simulink model "Main_model"  (R2021b)
settings: Solver=ode23t  StartTime=0.0  StopTime=sim_t_end  RelTol=1e-3
undefined symbols (not defined in the file): ambient_co2, ambient_pressure, ambient_rh, ambient_temp, battery, battery_heat_gen_scale, battery_mass, battery_thermal_mass, cab_air_v_dot, cabin_heater_cmd, cabin_heater_max_power, case_cold_plate_mass, case_cold_plate_thermal_mass, chiller_baffles_n, chiller_tube_length, chiller_tubes_n_rows, compressor_max_m_dot, compressor_ref_m_dot, condenser_air_min_flow_area, condenser_tube_width, const_current, coolant_channel_length, coolant_initial_T, coolant_m_dot, coolant_pipe_cross_sec_area, evaporator_air_cross_sec_area, evaporator_air_min_flow_area, evaporator_tube_width, motor_mc_heat_fraction, n_parallel, power_fraction_rear, ptc_heater_max_power, ptc_heater_thermal_mass, rad_air_v_dot, radiator_air_cross_sec_area, radiator_air_min_flow_area, radiator_tube_width, ref_m_dot, ref_pipe_dia, refrigerant_initial_void_fraction, refrigerant_pipe_cross_sec_area, T_bat_active_cool, T_bat_active_heat, T_bat_passive_cool, T_bat_passive_heat, T_battery_init, T_battery_nom, T_cabin_init, T_cabin_setpoint, T_dcdc_nom, T_DT_high, T_DT_passive_cool, T_DT_whr_active, T_front_gb_nom, T_front_mc_nom, T_front_motor_nom, T_rear_gb_nom, T_rear_mc_nom, T_rear_motor_nom, three_w_valve_max_open_area_factor ... (+3)
libraries: fl_lib x448, nesl_utility x328, SimscapeFluids_lib x134, slpidlib x15, ee_lib x9, simulink x8, LiBatteryElements_lib x4, SignalEditorBlockLib x1
(part 11 of 24)

== system Main_model/HVAC cycles/4 Way Valve (2P)2 ==
  Orifice (2P){6..9} (4 alike) : SimscapeFluids_lib/Two-Phase Fluid/Valves & Orifices/Orifice (2P)  orifice_type=foundation.enum.constant_variable.variable  mdot_nominal_constant=0.1 kg/s  delta_p_nominal_constant=0.001 MPa  S_min=0 m  del_S=5e-3 m  open_orientation=fluids.two_phase_fluid.valves_orifices.enum.OrificeOrientation.Positive  mdot_nominal_max=0.018 kg/s  delta_p_nominal_max=0.001 MPa  energy_spec=foundation.enum.energy_spec.void_fraction  p_inlet=.7 MPa  T_inlet=293.15 K  x_inlet=0.5  alpha_inlet=refrigerant_initial_void_fraction  h_inlet=1500 kJ/kg  u_inlet=1500 kJ/kg  area=refrigerant_pipe_cross_sec_area m^2  mdot_leak_fraction=1e-6  smoothing_factor=0.01  B_lam=0.999  tau_x=0.1 s
      settings: SourceProductBaseCode=SH  InternalSimscapePortConfiguration="{\"Bottom\":[],\"Left\":[{\"id\":\"A\",\"label\":\"A\",\"type\":\"foundation.two_phase_fluid.two_phase_fluid\"},{\"id\":\"S\",\"label\":\"S\",\"type\":\"input\"}],\"Right\":[{\"id\":\"B\",\"label\":\"B\",\"type\":\"foundation.two_phase_fluid.two_phase_fluid\"}],\"Top\":[]}"
  PS Gain : fl_lib/Physical Signals/Functions/PS Gain  gain=-1
  Simulink-PS Converter : nesl_utility/Simulink-PS Converter  PhysicalDomain=network_engine_domain  SubClassName=ps_input  LeftPortType=input  RightPortType=output  PseudoPeriodic=off  Frequencies=[]  NoiseDistribution=none  NoiseParameters=[]  Unit=1  AffineConversion=off  FilteringAndDerivatives=provide  SimscapeFilterOrder=1  InputFilterTimeConstant=0.001  UdotUserProvided=0
      settings: SourceProductBaseCode=PW,SS
  A1 : PMIOPort  Side=Left
  A2 : PMIOPort  Port=2  Side=Right
  B2 : PMIOPort  Port=3  Side=Left
  B1 : PMIOPort  Port=4  Side=Right
  wires:
  [cmd_cool_heat_loop] -> Simulink-PS Converter/1
  connections:
  B2/RConn1 -- Orifice (2P)8/LConn1 -- Orifice (2P)9/RConn1
  Orifice (2P)9/LConn2 -- PS Gain/LConn1 -- Orifice (2P)6/LConn2 -- Simulink-PS Converter/RConn1
  A2/RConn1 -- Orifice (2P)7/LConn1 -- Orifice (2P)6/RConn1
  A1/RConn1 -- Orifice (2P)6/LConn1 -- Orifice (2P)8/RConn1
  B1/RConn1 -- Orifice (2P)7/RConn1 -- Orifice (2P)9/LConn1
  Orifice (2P)8/LConn2 -- PS Gain/RConn1 -- Orifice (2P)7/LConn2

== system Main_model/HVAC cycles/4 Way Valve (2P)3 ==
  Orifice (2P){6..9} (4 alike) : SimscapeFluids_lib/Two-Phase Fluid/Valves & Orifices/Orifice (2P)  orifice_type=foundation.enum.constant_variable.variable  mdot_nominal_constant=0.1 kg/s  delta_p_nominal_constant=0.001 MPa  S_min=0 m  del_S=5e-3 m  open_orientation=fluids.two_phase_fluid.valves_orifices.enum.OrificeOrientation.Positive  mdot_nominal_max=0.018 kg/s  delta_p_nominal_max=0.001 MPa  energy_spec=foundation.enum.energy_spec.void_fraction  p_inlet=.7 MPa  T_inlet=293.15 K  x_inlet=0.5  alpha_inlet=refrigerant_initial_void_fraction  h_inlet=1500 kJ/kg  u_inlet=1500 kJ/kg  area=refrigerant_pipe_cross_sec_area m^2  mdot_leak_fraction=1e-6  smoothing_factor=0.01  B_lam=0.999  tau_x=0.1 s
      settings: SourceProductBaseCode=SH  InternalSimscapePortConfiguration="{\"Bottom\":[],\"Left\":[{\"id\":\"A\",\"label\":\"A\",\"type\":\"foundation.two_phase_fluid.two_phase_fluid\"},{\"id\":\"S\",\"label\":\"S\",\"type\":\"input\"}],\"Right\":[{\"id\":\"B\",\"label\":\"B\",\"type\":\"foundation.two_phase_fluid.two_phase_fluid\"}],\"Top\":[]}"
  PS Gain : fl_lib/Physical Signals/Functions/PS Gain  gain=-1
  Simulink-PS Converter : nesl_utility/Simulink-PS Converter  PhysicalDomain=network_engine_domain  SubClassName=ps_input  LeftPortType=input  RightPortType=output  PseudoPeriodic=off  Frequencies=[]  NoiseDistribution=none  NoiseParameters=[]  Unit=1  AffineConversion=off  FilteringAndDerivatives=provide  SimscapeFilterOrder=1  InputFilterTimeConstant=0.001  UdotUserProvided=0
      settings: SourceProductBaseCode=PW,SS
  A1 : PMIOPort  Side=Left
  A2 : PMIOPort  Port=2  Side=Right
  B2 : PMIOPort  Port=3  Side=Left
  B1 : PMIOPort  Port=4  Side=Right
  wires:
  [cmd_cool_heat_loop] -> Simulink-PS Converter/1
  connections:
  B2/RConn1 -- Orifice (2P)8/LConn1 -- Orifice (2P)9/RConn1
  Orifice (2P)9/LConn2 -- PS Gain/LConn1 -- Orifice (2P)6/LConn2 -- Simulink-PS Converter/RConn1
  A2/RConn1 -- Orifice (2P)7/LConn1 -- Orifice (2P)6/RConn1
  A1/RConn1 -- Orifice (2P)6/LConn1 -- Orifice (2P)8/RConn1
  B1/RConn1 -- Orifice (2P)7/RConn1 -- Orifice (2P)9/LConn1
  Orifice (2P)8/LConn2 -- PS Gain/RConn1 -- Orifice (2P)7/LConn2

== system Main_model/HVAC cycles/Compressor On-Off ==
  1-D Lookup Table : Lookup_n-D  NumberOfTableDimensions=1  BreakpointsForDimension1=[0,.03,0.05,0.1,0.15,0.2,0.25,0.3,1]  Table=[0,0,0.1*compressor_ref_m_dot,0.3*compressor_ref_m_dot,0.4*compressor_ref_m_dot,0.5*compressor_ref_m_dot,0.7*compressor_ref_m_dot,compressor_ref_m_dot,compressor_ref_m_dot]  InternalRulePriority=Speed  RndMeth=Simplest  InputSameDT=on
  1-D Lookup Table1 : Lookup_n-D  NumberOfTableDimensions=1  BreakpointsForDimension1=[0.5,0.7,1,2,3,4,5,5.5]  Table=[compressor_ref_m_dot,compressor_ref_m_dot,compressor_ref_m_dot,.7*compressor_ref_m_dot,.2*compressor_ref_m_dot,.005*compressor_ref_m_dot,0,0]  InternalRulePriority=Speed  RndMeth=Simplest  InputSameDT=on
  Constant : Constant  Value=ambient_temp
  Constant1 : Constant  Commented=on  Value=.0001
  Constant2 : Constant  Value=T_cabin_setpoint
  Constant3 : Constant  Value=0
  Constant4 : Constant  Commented=on  Value=.05
  Constant5 : Constant
  Constant6 : Constant  Value=0
  Constant7 : Constant  Value=-1
  Constant8 : Constant
  Data Type Conversion1 : DataTypeConversion
  Data Type Conversion3 : DataTypeConversion
  Data Type Conversion4 : DataTypeConversion  Commented=on
  Delay : Delay  Commented=on  DelayLength=10
  Delay1 : Delay  Commented=on  DelayLength=10
  Gain : Gain  Gain=1/compressor_ref_m_dot
  Gain1 : Gain  Gain=60*5/18
  GreaterThan : RelationalOperator  Commented=on  Operator=>  OutDataTypeStr=boolean  RndMeth=Simplest
  GreaterThan1 : RelationalOperator  Operator=>  OutDataTypeStr=boolean  RndMeth=Simplest
  GreaterThan2 : RelationalOperator  Operator=<  OutDataTypeStr=boolean  RndMeth=Simplest
  GreaterThan3 : RelationalOperator  Operator=>  OutDataTypeStr=boolean  RndMeth=Simplest
  Min : MinMax  Inputs=2
  Mux : Mux  Inputs=2
  Mux1 : Mux  Inputs=3
  Relay1 : Relay  OnSwitchValue=T_cabin_setpoint+2  OffSwitchValue=T_cabin_setpoint-2  OnOutputValue=1.1*T_cabin_setpoint  OffOutputValue=0.9*T_cabin_setpoint
  Relay2 : Relay  OnSwitchValue=T_cabin_setpoint+2  OffSwitchValue=T_cabin_setpoint-2  OnOutputValue=1.1*T_cabin_setpoint  OffOutputValue=0.9*T_cabin_setpoint
  Scope : Scope  NumInputPorts=2
  Scope2 : Scope  NumInputPorts=2
  Step : Step  SampleTime=0
  Step1 : Step  SampleTime=0
  Switch{1..3,5} (4 alike) : Switch  Criteria=u2 > Threshold  OutDataTypeStr=double
  Switch4 : Switch  Commented=on  Criteria=u2 > Threshold  OutDataTypeStr=double
  Transfer Fcn1 : TransferFcn  Commented=on  Denominator=[.1 1]
  Transfer Fcn2 : TransferFcn  Denominator=[.5 1]
  tag scope: ac_onoff=global, cmd_compressor_m_dot=global, cmd_cool_heat_loop=global, cmd_hvac_pump_on_off=global, hvac_cmd_fan=global, veh_speed_m_s=global
  wires:
  Data Type Conversion1/1 -> Switch5/2, Switch1/2
  GreaterThan1/1 -> Switch2/1
  Constant3/1 -> Switch1/3
  Constant2/1 -> GreaterThan3/2, Mux1/2, GreaterThan1/2, GreaterThan2/2  "T setpoint"
  Switch2/1 -> Data Type Conversion1/1
  Constant/1 -> Mux1/3, GreaterThan3/1  "T ambient"
  GreaterThan2/1 -> Switch2/3
  GreaterThan3/1 -> Data Type Conversion3/1, Switch2/2
  [T_cabin] -> Relay1/1, Delay1/1, Mux1/1, Relay2/1  "T cabin"
  Transfer Fcn2/1 -> GreaterThan/1, Scope2/1, [cmd_compressor_m_dot], Gain/1  "cmd_compressor_m_dot"
  1-D Lookup Table/1 -> Min/1
  1-D Lookup Table1/1 -> Min/2
  [p_evap_comp_in] -> 1-D Lookup Table/1
  [p_cond_comp_in] -> 1-D Lookup Table1/1
  Min/1 -> Transfer Fcn2/1, Switch1/1
  Switch3/1 -> Mux/1, [cmd_cool_heat_loop]  "cmd cooling (1) or heating (-1) mode (4-way valve)"
  Constant7/1 -> Switch3/3
  Data Type Conversion3/1 -> Switch3/1, Switch3/2
  Gain/1 -> Mux/2  "cmd compressor refrigerant mass flow rate"
  Mux/1 -> Scope/2
  Mux1/1 -> Scope/1
  Constant1/1 -> GreaterThan/2
  GreaterThan/1 -> Switch4/2, Data Type Conversion4/1
  Data Type Conversion4/1 -> Switch4/1
  Switch4/1 -> Scope2/2, Transfer Fcn1/1  "cmd_hvac_pump_on_off"
  Constant4/1 -> Switch4/3
  Constant5/1 -> [cmd_hvac_pump_on_off]  "cmd_compressor_m_dot"
  Constant6/1 -> Switch5/3
  Constant8/1 -> Switch5/1
  Switch5/1 -> [ac_onoff]
  Relay2/1 -> GreaterThan1/1
  Relay1/1 -> GreaterThan2/1
  Step/1 -> [hvac_cmd_fan]
  Gain1/1 -> [veh_speed_m_s]
  Step1/1 -> Gain1/1

== system Main_model/HVAC cycles/LCC4 ==
  lcc : SimscapeFluids_lib/Fluid Network Interfaces/Heat Exchangers/Condenser Evaporator (TL-2P)  flow_arrangement=fluids.interfaces.heat_exchangers.enum.FlowArrangementTL2P.Cross  cross_flow_arrangement=fluids.interfaces.heat_exchangers.enum.CrossFlowArrangementTL2P.UnmixedMixed  R_wall=chiller_wall_thermal_resistance K/kW  area_A1=coolant_pipe_cross_sec_area m^2  area_B1=coolant_pipe_cross_sec_area m^2  area_A2=refrigerant_pipe_cross_sec_area m^2  area_B2=refrigerant_pipe_cross_sec_area m^2  flow_geometry_TL=fluids.interfaces.heat_exchangers.enum.FlowGeometryTL.AcrossTubeBank  tube_num_TL=25  tube_length_TL=1 m  tube_cross_section_TL=fluids.interfaces.heat_exchangers.enum.TubeCrossSection.Rectangular  tube_diameter_TL=0.05 m  tube_width_TL=.02 m  tube_height_TL=0.003 m  tube_inner_diameter_TL=0.05 m  tube_outer_diameter_TL=0.1 m  tube_flow_area_TL=0.002 m^2  tube_wetted_perimeter_TL=0.15 m  tube_heat_perimeter_TL=0.15 m  tube_pressure_loss_spec_TL=fluids.interfaces.heat_exchangers.enum.TubePressureLossSpec.Haaland  tube_loss_coeff_TL=10  tube_length_add_TL=4 m  tube_roughness_pressure_TL=15e-6 m  tube_Re_lam_pressure_TL=2000  tube_Re_tur_pressure_TL=4000  tube_shape_factor_generic_TL=64  tube_heat_coeff_spec_TL=fluids.interfaces.heat_exchangers.enum.TubeHeatCoeffSpec.Gneilinski  tube_colburn_coeff_TL=[.023, .8, .33]  tube_roughness_heat_TL=15e-6 m  tube_Re_lam_heat_TL=2000  tube_Re_tur_heat_TL=4000  tube_Nu_lam_generic_TL=3.66  bank_arrangement_TL=fluids.interfaces.heat_exchangers.enum.BankArrangement.Staggered  bank_num_rows_TL=chiller_tubes_n_rows*(chiller_baffles_n+1)  bank_tubes_per_row_TL=chiller_tubes_n_columns  bank_width_TL=chiller_tube_length/(chiller_baffles_n+1) m  bank_tube_diameter_TL=chiller_tube_dia m  bank_longitudinal_pitch_TL=chiller_long_pitch m  bank_transverse_pitch_TL=chiller_transverse_pitch m  bank_pressure_loss_spec_TL=fluids.interfaces.heat_exchangers.enum.BankPressureLossSpec.Euler  bank_euler_TL=70  bank_heat_coeff_spec_TL=fluids.interfaces.heat_exchangers.enum.BankHeatCoeffSpec.Colburn  bank_colburn_coeff_TL=[0.27, .67, 0.36]  generic_flow_area_TL=0.01 m^2  generic_heat_area_TL=2 m^2  generic_volume_TL=0.05 m^3  generic_loss_coeff_TL=10  generic_colburn_coeff_TL=[.023, .8, .33]  fouling_factor_TL=0.1 K*m^2/kW  fin_area_TL=chiller_baffles_area m^2  fin_efficiency_TL=chiller_bafffles_fin_eff  p_init_TL=ambient_pressure MPa  T_init_TL=ambient_temp K  tube_num_2P=chiller_tubes_n_total  tube_length_2P=chiller_tube_length m  tube_cross_section_2P=fluids.interfaces.heat_exchangers.enum.TubeCrossSection.Circular  tube_diameter_2P=chiller_tube_dia m  tube_width_2P=0.05 m  tube_height_2P=0.05 m  tube_inner_diameter_2P=0.05 m  tube_outer_diameter_2P=0.1 m  tube_flow_area_2P=0.002 m^2  tube_wetted_perimeter_2P=0.15 m  tube_heat_perimeter_2P=0.15 m  tube_pressure_loss_spec_2P=fluids.interfaces.heat_exchangers.enum.TubePressureLossSpec2P.LossCoeff  tube_loss_coeff_2P=10  tube_length_add_2P=chiller_tube_eqv_resistance_length m  tube_roughness_pressure_2P=15e-6 m  tube_Re_lam_pressure_2P=2000  tube_Re_tur_pressure_2P=4000  tube_shape_factor_generic_2P=64  tube_heat_coeff_spec_2P=fluids.interfaces.heat_exchangers.enum.TubeHeatCoeffSpec2P.Colburn  tube_colburn_coeff_liq_2P=[0.27, .67, 0.36]  tube_colburn_coeff_mix_2P=[0.27, .67, 0.36]  tube_colburn_coeff_vap_2P=[0.27, .67, 0.36]  tube_roughness_heat_2P=15e-6 m  tube_Re_lam_heat_2P=2000  tube_Re_tur_heat_2P=4000  tube_Nu_lam_generic_2P=3.66  fouling_factor_2P=0.1 K*m^2/kW  fin_area_2P=0 m^2  fin_efficiency_2P=0  energy_spec_2P=foundation.enum.energy_spec.void_fraction  p_init_2P=refrigerant_initial_P MPa  T_init_2P=refrigerant_initial_T K  x_init_2P=0.5  alpha_init_2P=refrigerant_initial_void_fraction  h_init_2P=1500 kJ/kg  u_init_2P=1500 kJ/kg
      settings: SourceProductBaseCode=SH  InternalSimscapePortConfiguration="{\"Bottom\":[],\"Left\":[{\"id\":\"A1\",\"label\":\"A1\",\"type\":\"foundation.thermal_liquid.thermal_liquid\"},{\"id\":\"B1\",\"label\":\"B1\",\"type\":\"foundation.thermal_liquid.thermal_liquid\"}],\"Right\":[{\"id\":\"A2\",\"label\":\"A2\",\"type\":\"foundation.two_phase_fluid.two_phase_fluid\"},{\"id\":\"B2\",\"label\":\"B2\",\"type\":\"foundation.two_phase_fluid.two_phase_fluid\"}],\"Top\":[{\"id\":\"Z\",\"label\":\"Z\",\"type\":\"output\"}]}"
  Coolant Out : PMIOPort  Side=Left
  Coolant In : PMIOPort  Port=2  Side=Left
  Ref In : PMIOPort  Port=3  Side=Right
  Ref Out : PMIOPort  Port=4  Side=Right
  connections:
  lcc/RConn1 -- Ref In/RConn1
  lcc/LConn1 -- Coolant In/RConn1
  lcc/LConn2 -- Coolant Out/RConn1
  lcc/RConn2 -- Ref Out/RConn1

== system Main_model/HVAC cycles/TXV1 ==
  Cap (2P) : fl_lib/Two-Phase Fluid/Elements/Cap (2P)  p_specify=off  p_priority=None  p=0.101325 MPa  p_nominal_specify=off  p_nominal_unit=MPa  p_nominal_value=1  u_specify=off  u_priority=None  u=1.5e+3 kJ/kg  u_nominal_specify=off  u_nominal_unit=kJ/kg  u_nominal_value=1
      settings: SourceProductBaseCode=SS  InternalSimscapePortConfiguration="{\"Bottom\":[],\"Left\":[{\"id\":\"A\",\"label\":\"\",\"type\":\"foundation.two_phase_fluid.two_phase_fluid\"}],\"Right\":[],\"Top\":[]}"
  Cap (2P)1 : fl_lib/Two-Phase Fluid/Elements/Cap (2P)  p_specify=off  p_priority=None  p=0.101325 MPa  p_nominal_specify=off  p_nominal_unit=MPa  p_nominal_value=1  u_specify=off  u_priority=None  u=1.5e+3 kJ/kg  u_nominal_specify=off  u_nominal_unit=kJ/kg  u_nominal_value=1
      settings: SourceProductBaseCode=SS  InternalSimscapePortConfiguration="{\"Bottom\":[],\"Left\":[{\"id\":\"A\",\"label\":\"\",\"type\":\"foundation.two_phase_fluid.two_phase_fluid\"}],\"Right\":[],\"Top\":[]}"
  Expansion Valve : SimscapeFluids_lib/Two-Phase Fluid/Valves & Orifices/Flow Control Valves/Thermostatic Expansion Valve (2P)  Q_nominal=txv_nom_capacity W  Q_max=txv_max_capacity W  T_evap=evap_nom_temp K  delta_T_static=evap_min_superheat_delta deltaK  delta_T_nominal=evap_nom_superheat_delta deltaK  T_cond=cond_nom_temp K  delta_T_sub=cond_nom_subcool_delta deltaK  pressure_equalization=fluids.two_phase_fluid.valves_orifices.flow_control_valves.enum.ThermostaticExpansionValveEqualization.External  mop=fluids.two_phase_fluid.valves_orifices.flow_control_valves.enum.ThermostaticExpansionValveMOP.Pressure  p_mop=0.5 MPa  T_mop=288.15 K  bulb_dynamics=simscape.enum.onoff.off  tau_bulb=20 s  area=refrigerant_pipe_cross_sec_area m^2  mdot_leak_fraction=1e-6  smoothing_factor=0.01  B_lam=0.999  tau_x=0.1 s
      settings: SourceProductBaseCode=SH  InternalSimscapePortConfiguration="{\"Bottom\":[],\"Left\":[{\"id\":\"A\",\"label\":\"A\",\"type\":\"foundation.two_phase_fluid.two_phase_fluid\"}],\"Right\":[{\"id\":\"B\",\"label\":\"B\",\"type\":\"foundation.two_phase_fluid.two_phase_fluid\"}],\"Top\":[{\"id\":\"S\",\"label\":\"S\",\"type\":\"foundation.two_phase_fluid.two_phase_fluid\"},{\"id\":\"E\",\"label\":\"E\",\"type\":\"foundation.two_phase_fluid.two_phase_fluid\"}]}"
  Gain : Gain  Gain=-1
  Orifice (2P){1..3,7} (4 alike) : SimscapeFluids_lib/Two-Phase Fluid/Valves & Orifices/Orifice (2P)  orifice_type=foundation.enum.constant_variable.variable  mdot_nominal_constant=0.1 kg/s  delta_p_nominal_constant=0.001 MPa  S_min=0 m  del_S=5e-3 m  open_orientation=fluids.two_phase_fluid.valves_orifices.enum.OrificeOrientation.Positive  mdot_nominal_max=0.018 kg/s  delta_p_nominal_max=0.001 MPa  energy_spec=foundation.enum.energy_spec.void_fraction  p_inlet=.7 MPa  T_inlet=293.15 K  x_inlet=0.5  alpha_inlet=refrigerant_initial_void_fraction  h_inlet=1500 kJ/kg  u_inlet=1500 kJ/kg  area=refrigerant_pipe_cross_sec_area m^2  mdot_leak_fraction=1e-6  smoothing_factor=0.01  B_lam=0.999  tau_x=0.1 s
      settings: SourceProductBaseCode=SH  InternalSimscapePortConfiguration="{\"Bottom\":[],\"Left\":[{\"id\":\"A\",\"label\":\"A\",\"type\":\"foundation.two_phase_fluid.two_phase_fluid\"},{\"id\":\"S\",\"label\":\"S\",\"type\":\"input\"}],\"Right\":[{\"id\":\"B\",\"label\":\"B\",\"type\":\"foundation.two_phase_fluid.two_phase_fluid\"}],\"Top\":[]}"
  Perfect Insulator : fl_lib/Thermal/Thermal Elements/Perfect Insulator  T_specify=off  T_priority=None  T=0 K  T_nominal_specify=off  T_nominal_unit=K  T_nominal_value=1
  Receiver : SimscapeFluids_lib/Two-Phase Fluid/Tanks & Accumulators/Receiver Accumulator (2P)  volume=refrigerant_tank_vol l  area_AV=0.01 m^2  area_BV=0.01 m^2  area_AL=refrigerant_pipe_cross_sec_area m^2  area_BL=refrigerant_pipe_cross_sec_area m^2  V_frac_error=simscape.enum.assert.action.none  V_frac_min=0.05  V_frac_max=0.95  V_frac_smooth=0.05  p_crit_error=simscape.enum.assert.action.warn  hc_vap=20 W/(m^2*K)  hc_liq=100 W/(m^2*K)  surface_area=0.1 m^2  receiver_accumulator_energy_spec=fluids.two_phase_fluid.enum.receiver_accumulator_energy_spec.volume_fraction  p_init=refrigerant_initial_P MPa  T_init=293.15 K  M_frac_init=0.5  V_frac_init=1-refrigerant_initial_void_fraction  h_init=1500 kJ/kg  u_init=1500 kJ/kg  tau_vap_cond=1 s
      settings: SourceProductBaseCode=SH  InternalSimscapePortConfiguration="{\"Bottom\":[],\"Left\":[{\"id\":\"AV\",\"label\":\"AV\",\"type\":\"foundation.two_phase_fluid.two_phase_fluid\"},{\"id\":\"AL\",\"label\":\"AL\",\"type\":\"foundation.two_phase_fluid.two_phase_fluid\"},{\"id\":\"H\",\"label\":\"H\",\"type\":\"foundation.thermal.thermal\"}],\"Right\":[{\"id\":\"BV\",\"label\":\"BV\",\"type\":\"foundation.two_phase_fluid.two_phase_fluid\"},{\"id\":\"BL\",\"label\":\"BL\",\"type\":\"foundation.two_phase_fluid.two_phase_fluid\"},{\"id\":\"L\",\"label\":\"L\",\"type\":\"output\"}],\"Top\":[]}"
  Simulink-PS Converter{,1..3} (4 alike) : nesl_utility/Simulink-PS Converter  PhysicalDomain=network_engine_domain  SubClassName=ps_input  LeftPortType=input  RightPortType=output  PseudoPeriodic=off  Frequencies=[]  NoiseDistribution=none  NoiseParameters=[]  Unit=1  AffineConversion=off  FilteringAndDerivatives=provide  SimscapeFilterOrder=1  InputFilterTimeConstant=0.001  UdotUserProvided=0
      settings: SourceProductBaseCode=PW,SS
  Solver Configuration : nesl_utility/Solver Configuration  PhysicalDomain=network_engine_domain  SubClassName=solver  LeftPortType=input  RightPortType=generic  Tones=[]  Harmonics=[]  SimulateNoise=off  Profile=off  UseLocalSampling=off  EnableSwitchedLinearOptims=on  FrequencyDomain=off  UseCCode=off  RelTol=0.001  AbsTol=1e-06  MinStep=1e-09  ToWorkspace=off  RevertToSquareIcSolve=off  NumHomotopyIterations=100  PhasorMode=off  PhasorModeNumHarmonics=1  DoDC=off  ResidualTolerance=1e-09  UseLocalSolver=off  LocalSolverChoice=NE_BACKWARD_EULER_ADVANCER  LocalSolverSampleTime=0.001  DoFixedCost=off  MaxNonlinIter=3  MaxModeIter=2  ComputeImpulses=off  ImpulseIterations=2  LinearAlgebra=auto  EquationFormulation=NE_TIME_EF  DelaysMemoryBudget=1024  AutomaticFiltering=on  FilteringTimeConstant=0.001  PartitionStorageMethod=AS_NEEDED  PartitionMemoryBudget=1024  PartitionMethod=ROBUST
      settings: SourceProductBaseCode=PW,SS
  Thermodynamic Properties Sensor (2P) : fl_lib/Two-Phase Fluid/Sensors/Thermodynamic Properties Sensor (2P)
      settings: SourceProductBaseCode=SS  InternalSimscapePortConfiguration="{\"Bottom\":[],\"Left\":[{\"id\":\"A\",\"label\":\"A\",\"type\":\"foundation.two_phase_fluid.two_phase_fluid\"}],\"Right\":[{\"id\":\"T\",\"label\":\"T\",\"type\":\"output\"},{\"id\":\"H\",\"label\":\"h\",\"type\":\"output\"},{\"id\":\"V\",\"label\":\"v\",\"type\":\"output\"},{\"id\":\"S\",\"label\":\"s\",\"type\":\"output\"}],\"Top\":[]}"
  heat loss : Subsystem
  Ref In : PMIOPort  Side=Left
  Ref Out : PMIOPort  Port=2  Side=Left
  "Bulb " : PMIOPort  Port=3  Side=Left
  wires:
  Gain/1 -> Simulink-PS Converter1/1, Simulink-PS Converter/1
  [cmd_cool_heat_loop] -> Simulink-PS Converter3/1, Simulink-PS Converter2/1, Gain/1
  connections:
  "Bulb "/RConn1 -- Expansion Valve/LConn2 -- Expansion Valve/LConn3
  Orifice (2P)1/LConn1 -- Orifice (2P)3/LConn1 -- Ref In/RConn1
  Perfect Insulator/LConn1 -- Receiver/LConn3
  Cap (2P)1/LConn1 -- Receiver/RConn1
  Cap (2P)/LConn1 -- Receiver/LConn1
  Expansion Valve/LConn1 -- Receiver/RConn2
  Simulink-PS Converter/RConn1 -- Orifice (2P)7/LConn2
  Orifice (2P)7/RConn1 -- Orifice (2P)2/RConn1 -- Ref Out/RConn1
  Simulink-PS Converter1/RConn1 -- Orifice (2P)1/LConn2
  Simulink-PS Converter2/RConn1 -- Orifice (2P)2/LConn2
  Orifice (2P)1/RConn1 -- Solver Configuration/RConn1 -- Receiver/LConn2 -- Orifice (2P)2/LConn1
  Simulink-PS Converter3/RConn1 -- Orifice (2P)3/LConn2
  Expansion Valve/RConn1 -- Thermodynamic Properties Sensor (2P)/LConn1 -- heat loss/LConn1
  Orifice (2P)3/RConn1 -- heat loss/RConn1 -- Orifice (2P)7/LConn1

== system Main_model/HVAC cycles/TXV4 ==
  Cap (2P) : fl_lib/Two-Phase Fluid/Elements/Cap (2P)  p_specify=off  p_priority=None  p=0.101325 MPa  p_nominal_specify=off  p_nominal_unit=MPa  p_nominal_value=1  u_specify=off  u_priority=None  u=1.5e+3 kJ/kg  u_nominal_specify=off  u_nominal_unit=kJ/kg  u_nominal_value=1
      settings: SourceProductBaseCode=SS  InternalSimscapePortConfiguration="{\"Bottom\":[],\"Left\":[{\"id\":\"A\",\"label\":\"\",\"type\":\"foundation.two_phase_fluid.two_phase_fluid\"}],\"Right\":[],\"Top\":[]}"
  Cap (2P)1 : fl_lib/Two-Phase Fluid/Elements/Cap (2P)  p_specify=off  p_priority=None  p=0.101325 MPa  p_nominal_specify=off  p_nominal_unit=MPa  p_nominal_value=1  u_specify=off  u_priority=None  u=1.5e+3 kJ/kg  u_nominal_specify=off  u_nominal_unit=kJ/kg  u_nominal_value=1
      settings: SourceProductBaseCode=SS  InternalSimscapePortConfiguration="{\"Bottom\":[],\"Left\":[{\"id\":\"A\",\"label\":\"\",\"type\":\"foundation.two_phase_fluid.two_phase_fluid\"}],\"Right\":[],\"Top\":[]}"
  Expansion Valve : SimscapeFluids_lib/Two-Phase Fluid/Valves & Orifices/Flow Control Valves/Thermostatic Expansion Valve (2P)  Q_nominal=txv_nom_capacity W  Q_max=txv_max_capacity W  T_evap=evap_nom_temp K  delta_T_static=evap_min_superheat_delta deltaK  delta_T_nominal=evap_nom_superheat_delta deltaK  T_cond=cond_nom_temp K  delta_T_sub=cond_nom_subcool_delta deltaK  pressure_equalization=fluids.two_phase_fluid.valves_orifices.flow_control_valves.enum.ThermostaticExpansionValveEqualization.External  mop=fluids.two_phase_fluid.valves_orifices.flow_control_valves.enum.ThermostaticExpansionValveMOP.Pressure  p_mop=0.5 MPa  T_mop=288.15 K  bulb_dynamics=simscape.enum.onoff.off  tau_bulb=.1 s  area=refrigerant_pipe_cross_sec_area m^2  mdot_leak_fraction=1e-6  smoothing_factor=0.01  B_lam=0.999  tau_x=0.1 s
      settings: SourceProductBaseCode=SH  InternalSimscapePortConfiguration="{\"Bottom\":[],\"Left\":[{\"id\":\"A\",\"label\":\"A\",\"type\":\"foundation.two_phase_fluid.two_phase_fluid\"}],\"Right\":[{\"id\":\"B\",\"label\":\"B\",\"type\":\"foundation.two_phase_fluid.two_phase_fluid\"}],\"Top\":[{\"id\":\"S\",\"label\":\"S\",\"type\":\"foundation.two_phase_fluid.two_phase_fluid\"},{\"id\":\"E\",\"label\":\"E\",\"type\":\"foundation.two_phase_fluid.two_phase_fluid\"}]}"
  Gain : Gain  Gain=-1
  Orifice (2P){1..3,7} (4 alike) : SimscapeFluids_lib/Two-Phase Fluid/Valves & Orifices/Orifice (2P)  orifice_type=foundation.enum.constant_variable.variable  mdot_nominal_constant=0.1 kg/s  delta_p_nominal_constant=0.001 MPa  S_min=0 m  del_S=5e-3 m  open_orientation=fluids.two_phase_fluid.valves_orifices.enum.OrificeOrientation.Positive  mdot_nominal_max=0.018 kg/s  delta_p_nominal_max=0.001 MPa  energy_spec=foundation.enum.energy_spec.void_fraction  p_inlet=.7 MPa  T_inlet=293.15 K  x_inlet=0.5  alpha_inlet=refrigerant_initial_void_fraction  h_inlet=1500 kJ/kg  u_inlet=1500 kJ/kg  area=refrigerant_pipe_cross_sec_area m^2  mdot_leak_fraction=1e-6  smoothing_factor=0.01  B_lam=0.999  tau_x=0.1 s
      settings: SourceProductBaseCode=SH  InternalSimscapePortConfiguration="{\"Bottom\":[],\"Left\":[{\"id\":\"A\",\"label\":\"A\",\"type\":\"foundation.two_phase_fluid.two_phase_fluid\"},{\"id\":\"S\",\"label\":\"S\",\"type\":\"input\"}],\"Right\":[{\"id\":\"B\",\"label\":\"B\",\"type\":\"foundation.two_phase_fluid.two_phase_fluid\"}],\"Top\":[]}"
  Perfect Insulator : fl_lib/Thermal/Thermal Elements/Perfect Insulator  T_specify=off  T_priority=None  T=0 K  T_nominal_specify=off  T_nominal_unit=K  T_nominal_value=1
  Receiver : SimscapeFluids_lib/Two-Phase Fluid/Tanks & Accumulators/Receiver Accumulator (2P)  volume=refrigerant_tank_vol l  area_AV=0.01 m^2  area_BV=0.01 m^2  area_AL=refrigerant_pipe_cross_sec_area m^2  area_BL=refrigerant_pipe_cross_sec_area m^2  V_frac_error=simscape.enum.assert.action.none  V_frac_min=0.05  V_frac_max=0.95  V_frac_smooth=0.05  p_crit_error=simscape.enum.assert.action.warn  hc_vap=20 W/(m^2*K)  hc_liq=100 W/(m^2*K)  surface_area=0.1 m^2  receiver_accumulator_energy_spec=fluids.two_phase_fluid.enum.receiver_accumulator_energy_spec.volume_fraction  p_init=refrigerant_initial_P MPa  T_init=293.15 K  M_frac_init=0.5  V_frac_init=1-refrigerant_initial_void_fraction  h_init=1500 kJ/kg  u_init=1500 kJ/kg  tau_vap_cond=1 s
      settings: SourceProductBaseCode=SH  InternalSimscapePortConfiguration="{\"Bottom\":[],\"Left\":[{\"id\":\"AV\",\"label\":\"AV\",\"type\":\"foundation.two_phase_fluid.two_phase_fluid\"},{\"id\":\"AL\",\"label\":\"AL\",\"type\":\"foundation.two_phase_fluid.two_phase_fluid\"},{\"id\":\"H\",\"label\":\"H\",\"type\":\"foundation.thermal.thermal\"}],\"Right\":[{\"id\":\"BV\",\"label\":\"BV\",\"type\":\"foundation.two_phase_fluid.two_phase_fluid\"},{\"id\":\"BL\",\"label\":\"BL\",\"type\":\"foundation.two_phase_fluid.two_phase_fluid\"},{\"id\":\"L\",\"label\":\"L\",\"type\":\"output\"}],\"Top\":[]}"
  Simulink-PS Converter{,1..3} (4 alike) : nesl_utility/Simulink-PS Converter  PhysicalDomain=network_engine_domain  SubClassName=ps_input  LeftPortType=input  RightPortType=output  PseudoPeriodic=off  Frequencies=[]  NoiseDistribution=none  NoiseParameters=[]  Unit=1  AffineConversion=off  FilteringAndDerivatives=provide  SimscapeFilterOrder=1  InputFilterTimeConstant=0.001  UdotUserProvided=0
      settings: SourceProductBaseCode=PW,SS
  Solver Configuration : nesl_utility/Solver Configuration  PhysicalDomain=network_engine_domain  SubClassName=solver  LeftPortType=input  RightPortType=generic  Tones=[]  Harmonics=[]  SimulateNoise=off  Profile=off  UseLocalSampling=off  EnableSwitchedLinearOptims=on  FrequencyDomain=off  UseCCode=off  RelTol=0.001  AbsTol=1e-06  MinStep=1e-09  ToWorkspace=off  RevertToSquareIcSolve=off  NumHomotopyIterations=100  PhasorMode=off  PhasorModeNumHarmonics=1  DoDC=off  ResidualTolerance=1e-09  UseLocalSolver=off  LocalSolverChoice=NE_BACKWARD_EULER_ADVANCER  LocalSolverSampleTime=0.001  DoFixedCost=off  MaxNonlinIter=3  MaxModeIter=2  ComputeImpulses=off  ImpulseIterations=2  LinearAlgebra=auto  EquationFormulation=NE_TIME_EF  DelaysMemoryBudget=1024  AutomaticFiltering=on  FilteringTimeConstant=0.001  PartitionStorageMethod=AS_NEEDED  PartitionMemoryBudget=1024  PartitionMethod=ROBUST
      settings: SourceProductBaseCode=PW,SS
  Thermodynamic Properties Sensor (2P) : fl_lib/Two-Phase Fluid/Sensors/Thermodynamic Properties Sensor (2P)
      settings: SourceProductBaseCode=SS  InternalSimscapePortConfiguration="{\"Bottom\":[],\"Left\":[{\"id\":\"A\",\"label\":\"A\",\"type\":\"foundation.two_phase_fluid.two_phase_fluid\"}],\"Right\":[{\"id\":\"T\",\"label\":\"T\",\"type\":\"output\"},{\"id\":\"H\",\"label\":\"h\",\"type\":\"output\"},{\"id\":\"V\",\"label\":\"v\",\"type\":\"output\"},{\"id\":\"S\",\"label\":\"s\",\"type\":\"output\"}],\"Top\":[]}"
  heat loss : Subsystem
  Ref In : PMIOPort  Side=Left
  Ref Out : PMIOPort  Port=2  Side=Left
  "Bulb " : PMIOPort  Port=3  Side=Left
  wires:
  Gain/1 -> Simulink-PS Converter1/1, Simulink-PS Converter/1
  [cmd_cool_heat_loop] -> Simulink-PS Converter3/1, Simulink-PS Converter2/1, Gain/1
  connections:
  "Bulb "/RConn1 -- Expansion Valve/LConn2 -- Expansion Valve/LConn3
  Orifice (2P)1/LConn1 -- Orifice (2P)3/LConn1 -- Ref In/RConn1
  Perfect Insulator/LConn1 -- Receiver/LConn3
  Cap (2P)1/LConn1 -- Receiver/RConn1
  Cap (2P)/LConn1 -- Receiver/LConn1
  Expansion Valve/LConn1 -- Receiver/RConn2
  Simulink-PS Converter/RConn1 -- Orifice (2P)7/LConn2
  Orifice (2P)7/RConn1 -- Orifice (2P)2/RConn1 -- Ref Out/RConn1
  Simulink-PS Converter1/RConn1 -- Orifice (2P)1/LConn2
  Simulink-PS Converter2/RConn1 -- Orifice (2P)2/LConn2
  Orifice (2P)1/RConn1 -- Solver Configuration/RConn1 -- Receiver/LConn2 -- Orifice (2P)2/LConn1
  Simulink-PS Converter3/RConn1 -- Orifice (2P)3/LConn2
  Expansion Valve/RConn1 -- Thermodynamic Properties Sensor (2P)/LConn1 -- heat loss/LConn1
  Orifice (2P)3/RConn1 -- heat loss/RConn1 -- Orifice (2P)7/LConn1

== system Main_model/HVAC cycles/cabin HX4 ==
  Absolute Reference (MA)1 : fl_lib/Moist Air/Elements/Absolute Reference (MA)
      settings: SourceProductBaseCode=SS
  Air Flow Rate : Constant  Value=.1
  Air Flow Rate1 : Constant  Value=250*.00047
  Cabin Evaporator (MA-2P) : SimscapeFluids_lib/Fluid Network Interfaces/Heat Exchangers/Condenser Evaporator (2P-MA)  Commented=on  flow_arrangement=fluids.interfaces.heat_exchangers.enum.FlowArrangement2PMA.Cross  cross_flow_arrangement=fluids.interfaces.heat_exchangers.enum.CrossFlowArrangement2PMA.UnmixedMixed  R_wall=evaporator_wall_thermal_resistance K/W  area_A1=refrigerant_pipe_cross_sec_area m^2  area_B1=refrigerant_pipe_cross_sec_area m^2  area_A2=evaporator_air_cross_sec_area m^2  area_B2=evaporator_air_cross_sec_area m^2  tube_num_2P=evaporator_n_tubes  tube_length_2P=evaporator_tube_length m  tube_cross_section_2P=fluids.interfaces.heat_exchangers.enum.TubeCrossSection.Rectangular  tube_diameter_2P=.01 m  tube_width_2P=evaporator_tube_width m  tube_height_2P=evaporator_tube_height m  tube_inner_diameter_2P=0.05 m  tube_outer_diameter_2P=0.1 m  tube_flow_area_2P=0.002 m^2  tube_wetted_perimeter_2P=0.15 m  tube_heat_perimeter_2P=0.15 m  tube_pressure_loss_spec_2P=fluids.interfaces.heat_exchangers.enum.TubePressureLossSpec2P.Haaland  tube_loss_coeff_2P=10  tube_length_add_2P=evaporator_tube_eqv_resistance_length m  tube_roughness_pressure_2P=15e-6 m  tube_Re_lam_pressure_2P=2000  tube_Re_tur_pressure_2P=4000  tube_shape_factor_generic_2P=64  tube_heat_coeff_spec_2P=fluids.interfaces.heat_exchangers.enum.TubeHeatCoeffSpec2P.GneilinskiCavalliniZecchin  tube_colburn_coeff_liq_2P=[.023, .8, .33]  tube_colburn_coeff_mix_2P=[.05, .8, .33]  tube_colburn_coeff_vap_2P=[.023, .8, .33]  tube_roughness_heat_2P=15e-6 m  tube_Re_lam_heat_2P=2000  tube_Re_tur_heat_2P=4000  tube_Nu_lam_generic_2P=3.66  fouling_factor_2P=0.1 K*m^2/kW  fin_area_2P=0 m^2  fin_efficiency_2P=0  energy_spec_2P=foundation.enum.energy_spec.void_fraction  p_init_2P=refrigerant_initial_P MPa  T_init_2P=293.15 K  x_init_2P=0.5  alpha_init_2P=refrigerant_initial_void_fraction  h_init_2P=1500 kJ/kg  u_init_2P=1500 kJ/kg  flow_geometry_MA=fluids.interfaces.heat_exchangers.enum.FlowGeometryMA.AcrossTubeBank  tube_num_MA=25  tube_length_MA=1 m  tube_cross_section_MA=fluids.interfaces.heat_exchangers.enum.TubeCrossSection.Circular  tube_diameter_MA=0.05 m  tube_width_MA=0.05 m  tube_height_MA=0.05 m  tube_inner_diameter_MA=0.05 m  tube_outer_diameter_MA=0.1 m  tube_flow_area_MA=0.002 m^2  tube_wetted_perimeter_MA=0.15 m  tube_heat_perimeter_MA=0.15 m  tube_pressure_loss_spec_MA=fluids.interfaces.heat_exchangers.enum.TubePressureLossSpec.Haaland  tube_loss_coeff_MA=10  tube_length_add_MA=0.1 m  tube_roughness_pressure_MA=15e-6 m  tube_Re_lam_pressure_MA=2000  tube_Re_tur_pressure_MA=4000  tube_shape_factor_generic_MA=64  tube_heat_coeff_spec_MA=fluids.interfaces.heat_exchangers.enum.TubeHeatCoeffSpec.Gneilinski  tube_colburn_coeff_MA=[.023, .8, .33]  tube_roughness_heat_MA=15e-6 m  tube_Re_lam_heat_MA=2000  tube_Re_tur_heat_MA=4000  tube_Nu_lam_generic_MA=3.66  bank_arrangement_MA=fluids.interfaces.heat_exchangers.enum.BankArrangement.Inline  bank_num_rows_MA=1  bank_tubes_per_row_MA=evaporator_n_tubes  bank_width_MA=evaporator_tube_length m  bank_tube_diameter_MA=evaporator_tube_height m  bank_longitudinal_pitch_MA=evaporator_tube_pitch m  bank_transverse_pitch_MA=evaporator_tube_pitch m  bank_pressure_loss_spec_MA=fluids.interfaces.heat_exchangers.enum.BankPressureLossSpec.Martin  bank_euler_MA=10  bank_heat_coeff_spec_MA=fluids.interfaces.heat_exchangers.enum.BankHeatCoeffSpec.Martin  bank_colburn_coeff_MA=[.27, .63, .36]  generic_flow_area_MA=evaporator_air_min_flow_area m^2  generic_heat_area_MA=evaporator_ht_surf_area_without_fins m^2  generic_volume_MA=evaporator_air_min_flow_area*evaporator_tube_width m^3  generic_loss_coeff_MA=10  generic_colburn_coeff_MA=[0.27, 0.63, 0.36]  fouling_factor_MA=0.1 K*m^2/kW  fin_area_MA=evaporator_fin_surf_area m^2  fin_efficiency_MA=evaporator_air_fin_eff  p_init_MA=ambient_pressure MPa  T_init_MA=ambient_temp K  moisture_spec_MA=foundation.enum.moisture_spec.relative_humidity  RH_init_MA=ambient_rh  x_w_init_MA=0.01  y_w_init_MA=0.01  HR_init_MA=0.01  trace_gas_spec_MA=foundation.enum.trace_gas_spec.mole_fraction  x_g_init_MA=ambient_co2  y_g_init_MA=ambient_co2  RH_ws_MA=1
      settings: SourceProductBaseCode=SH  InternalSimscapePortConfiguration="{\"Bottom\":[],\"Left\":[{\"id\":\"A1\",\"label\":\"A1\",\"type\":\"foundation.two_phase_fluid.two_phase_fluid\"},{\"id\":\"Z\",\"label\":\"Z\",\"type\":\"output\"},{\"id\":\"B1\",\"label\":\"B1\",\"type\":\"foundation.two_phase_fluid.two_phase_fluid\"}],\"Right\":[{\"id\":\"A2\",\"label\":\"A2\",\"type\":\"foundation.moist_air.moist_air\"},{\"id\":\"W\",\"label\":\"W\",\"type\":\"output\"},{\"id\":\"B2\",\"label\":\"B2\",\"type\":\"foundation.moist_air.moist_air\"}],\"Top\":[]}"
  Constant : Constant  Value=T_cabin_setpoint
  Constant1 : Constant  Value=ambient_temp
  Controlled Volumetric Flow Rate Source (MA) : fl_lib/Moist Air/Sources/Controlled Volumetric Flow Rate Source (MA)  power_spec=foundation.enum.power_spec.none  volumetric_flow_conditions=foundation.enum.volumetric_flow_conditions.standard  p_std=ambient_pressure MPa  T_std=ambient_temp K  RH_std=ambient_rh  area_A=evaporator_air_cross_sec_area m^2  area_B=evaporator_air_cross_sec_area m^2
      settings: SourceProductBaseCode=SS  InternalSimscapePortConfiguration="{\"Bottom\":[],\"Left\":[{\"id\":\"A\",\"label\":\"A\",\"type\":\"foundation.moist_air.moist_air\"},{\"id\":\"V\",\"label\":\"V\",\"type\":\"input\"}],\"Right\":[{\"id\":\"B\",\"label\":\"B\",\"type\":\"foundation.moist_air.moist_air\"}],\"Top\":[]}"
  Max Flow [m^3/s] : Gain  Gain=234*.00047
  PID Controller : slpidlib/PID Controller  Controller=PI  Form=Ideal  TimeDomain=Continuous-time  UseExternalTs=off  SampleTime=-1  IntegratorMethod=Forward Euler  FilterMethod=Forward Euler  ControllerParametersSource=internal  P=20*1/50  I=1/4*25*1/150  D=0  UseFilter=on  N=100  TunerSelectOption=Transfer Function Based (PID Tuner App)  InitialConditionSource=internal  InitialConditionForIntegrator=0  InitialConditionForFilter=0  DifferentiatorICPrevScaledInput=0  ExternalReset=none  TrackingMode=off  Kt=1  LimitOutput=on  SatLimitsSource=internal  UpperSaturationLimit=1  LowerSaturationLimit=0  LinearizeAsGain=on  AntiWindupMode=back-calculation  Kb=1  POutMin=[]  POutMax=[]  IOutMin=[]  IOutMax=[]  DOutMin=[]  DOutMax=[]  NOutMin=[]  NOutMax=[]  SumOutMin=[]  SumOutMax=[]  SaturationOutMin=[]  SaturationOutMax=[]  PParamMin=[]  PParamMax=[]  IParamMin=[]  IParamMax=[]  DParamMin=[]  DParamMax=[]  NParamMin=[]  NParamMax=[]  KbParamMin=[]  KbParamMax=[]  KtParamMin=[]  KtParamMax=[]  KbOutMin=[]  KbOutMax=[]  KtOutMin=[]  KtOutMax=[]  IntegratorOutMin=[]  IntegratorOutMax=[]  FilterOutMin=[]  FilterOutMax=[]  SumI1OutMin=[]  SumI1OutMax=[]  SumI2OutMin=[]  SumI2OutMax=[]  SumI3OutMin=[]  SumI3OutMax=[]  SumI4OutMin=[]  SumI4OutMax=[]  SumDOutMin=[]  SumDOutMax=[]  DifferentiatorOutMin=[]  DifferentiatorOutMax=[]  FilterDiffOutCoefMin=[]  FilterDiffOutCoefMax=[]  ReciprocalOutMin=[]  ReciprocalOutMax=[]  SumDenOutMin=[]  SumDenOutMax=[]  SumNumOutMin=[]  SumNumOutMax=[]  DivideOutMin=[]  DivideOutMax=[]  UdiffTsProdOutMin=[]  UdiffTsProdOutMax=[]  NTsProdOutMin=[]  NTsProdOutMax=[]  UintegralTsProdOutMin=[]  UintegralTsProdOutMax=[]  UngainTsProdOutMin=[]  UngainTsProdOutMax=[]  IntegratorContinuousStateAttributes=''  IntegratorStateMustResolveToSignalObject=off  IntegratorRTWStateStorageClass=Auto  FilterContinuousStateAttributes=''  FilterStateMustResolveToSignalObject=off  FilterRTWStateStorageClass=Auto  ParallelPVariant=Passthrough  IdealPVariant=InternalParameters  IVariant=InternalParameters  DVariant=Disabled  IntegratorVariant=Continuous  SatVariant=Enabled  AWVariant=BackCalculation  PCopyVariant=Disabled  TRVariant=Disabled  FdbkBlocksVariant=Forward  IdealPFdbkVariant=Disabled  SatFdbkVariant=Disabled  DerivativeFilterVariant=Disabled  NVariant=Disabled  NCopyVariant=Disabled_SignalSpec  FilterICVariant=Disabled  IntegratorICVariant=InternalICs  ExternalResetVariant=Disabled  TRSumVariant=Passthrough  SumFdbkVariant=Disabled  SumVariant=Sum_PI  TsampFilterVariant=InternalTs  TsampNgainVariant=Passthrough  TsampIntegralVariant=Passthrough  ExternalSaturationOutDataTypeStr=Inherit: Same as second input
  PS-Simulink Converter4 : nesl_utility/PS-Simulink Converter  PhysicalDomain=network_engine_domain  SubClassName=ps_output  LeftPortType=input  RightPortType=output  PseudoPeriodic=off  Frequencies=[]  Unit=K  AffineConversion=off
      settings: SourceProductBaseCode=PW,SS
  Pressure & Temperature Sensor (MA)1 : fl_lib/Moist Air/Sensors/Pressure & Temperature Sensor (MA)
      settings: SourceProductBaseCode=SS  InternalSimscapePortConfiguration="{\"Bottom\":[],\"Left\":[{\"id\":\"A\",\"label\":\"A\",\"type\":\"foundation.moist_air.moist_air\"}],\"Right\":[{\"id\":\"B\",\"label\":\"B\",\"type\":\"foundation.moist_air.moist_air\"},{\"id\":\"P\",\"label\":\"P\",\"type\":\"output\"},{\"id\":\"T\",\"label\":\"T\",\"type\":\"output\"}],\"Top\":[]}"
  Product : Product
  Scope : Scope
  Sign : Signum
  Simulink-PS Converter9 : nesl_utility/Simulink-PS Converter  PhysicalDomain=network_engine_domain  SubClassName=ps_input  LeftPortType=input  RightPortType=output  PseudoPeriodic=off  Frequencies=[]  NoiseDistribution=none  NoiseParameters=[]  Unit=m^3/s  AffineConversion=off  FilteringAndDerivatives=provide  SimscapeFilterOrder=1  InputFilterTimeConstant=0.001  UdotUserProvided=0
      settings: SourceProductBaseCode=PW,SS
  Sum : Sum  Inputs=-+|
  Sum1 : Sum  Inputs=-+|
  Transfer Fcn : TransferFcn  Denominator=[5 1]
  cabin_hx : SimscapeFluids_lib/Fluid Network Interfaces/Heat Exchangers/Heat Exchanger (TL-MA)  flow_arrangement=fluids.interfaces.heat_exchangers.enum.FlowArrangementTLMA.Cross  cross_flow_arrangement=fluids.interfaces.heat_exchangers.enum.CrossFlowArrangementTLMA.UnmixedMixed  R_wall=evaporator_wall_thermal_resistance K/W  area_A1=coolant_pipe_cross_sec_area m^2  area_B1=coolant_pipe_cross_sec_area m^2  area_A2=evaporator_air_cross_sec_area m^2  area_B2=evaporator_air_cross_sec_area m^2  flow_geometry_TL=fluids.interfaces.heat_exchangers.enum.FlowGeometryTL.InsideTubes  tube_num_TL=evaporator_n_tubes  tube_length_TL=evaporator_tube_length m  tube_cross_section_TL=fluids.interfaces.heat_exchangers.enum.TubeCrossSection.Rectangular  tube_diameter_TL=0.05 m  tube_width_TL=evaporator_tube_width m  tube_height_TL=evaporator_tube_height m  tube_inner_diameter_TL=0.05 m  tube_outer_diameter_TL=0.1 m  tube_flow_area_TL=0.002 m^2  tube_wetted_perimeter_TL=0.15 m  tube_heat_perimeter_TL=0.15 m  tube_pressure_loss_spec_TL=fluids.interfaces.heat_exchangers.enum.TubePressureLossSpec.LossCoeff  tube_loss_coeff_TL=evaporator_coolant_pressure_loss_coef  tube_length_add_TL=evaporator_tube_eqv_resistance_length m  tube_roughness_pressure_TL=15e-6 m  tube_Re_lam_pressure_TL=2000  tube_Re_tur_pressure_TL=4000  tube_shape_factor_generic_TL=64  tube_heat_coeff_spec_TL=fluids.interfaces.heat_exchangers.enum.TubeHeatCoeffSpec.Colburn  tube_colburn_coeff_TL=[0.27, .67, 0.36]  tube_roughness_heat_TL=15e-6 m  tube_Re_lam_heat_TL=2000  tube_Re_tur_heat_TL=4000  tube_Nu_lam_generic_TL=3.66  bank_arrangement_TL=fluids.interfaces.heat_exchangers.enum.BankArrangement.Inline  bank_num_rows_TL=5  bank_tubes_per_row_TL=5  bank_width_TL=1 m  bank_tube_diameter_TL=0.05 m  bank_longitudinal_pitch_TL=0.15 m  bank_transverse_pitch_TL=0.15 m  bank_pressure_loss_spec_TL=fluids.interfaces.heat_exchangers.enum.BankPressureLossSpec.Martin  bank_euler_TL=10  bank_heat_coeff_spec_TL=fluids.interfaces.heat_exchangers.enum.BankHeatCoeffSpec.Martin  bank_colburn_coeff_TL=[.27, .63, .36]  generic_flow_area_TL=0.01 m^2  generic_heat_area_TL=2 m^2  generic_volume_TL=0.05 m^3  generic_loss_coeff_TL=10  generic_colburn_coeff_TL=[.023, .8, .33]  fouling_factor_TL=0 K*m^2/kW  fin_area_TL=0 m^2  fin_efficiency_TL=0  p_init_TL=coolant_initial_P MPa  T_init_TL=coolant_initial_T K  flow_geometry_MA=fluids.interfaces.heat_exchangers.enum.FlowGeometryMA.Generic  tube_num_MA=25  tube_length_MA=1 m  tube_cross_section_MA=fluids.interfaces.heat_exchangers.enum.TubeCrossSection.Circular  tube_diameter_MA=0.05 m  tube_width_MA=0.05 m  tube_height_MA=0.05 m  tube_inner_diameter_MA=0.05 m  tube_outer_diameter_MA=0.1 m  tube_flow_area_MA=0.002 m^2  tube_wetted_perimeter_MA=0.15 m  tube_heat_perimeter_MA=0.15 m  tube_pressure_loss_spec_MA=fluids.interfaces.heat_exchangers.enum.TubePressureLossSpec.Haaland  tube_loss_coeff_MA=10  tube_length_add_MA=0.1 m  tube_roughness_pressure_MA=15e-6 m  tube_Re_lam_pressure_MA=2000  tube_Re_tur_pressure_MA=4000  tube_shape_factor_generic_MA=64  tube_heat_coeff_spec_MA=fluids.interfaces.heat_exchangers.enum.TubeHeatCoeffSpec.Gneilinski  tube_colburn_coeff_MA=[.023, .8, .33]  tube_roughness_heat_MA=15e-6 m  tube_Re_lam_heat_MA=2000  tube_Re_tur_heat_MA=4000  tube_Nu_lam_generic_MA=3.66  bank_arrangement_MA=fluids.interfaces.heat_exchangers.enum.BankArrangement.Inline  bank_num_rows_MA=1  bank_tubes_per_row_MA=evaporator_n_tubes  bank_width_MA=evaporator_tube_length m  bank_tube_diameter_MA=evaporator_tube_height m  bank_longitudinal_pitch_MA=evaporator_tube_pitch m  bank_transverse_pitch_MA=evaporator_tube_pitch m  bank_pressure_loss_spec_MA=fluids.interfaces.heat_exchangers.enum.BankPressureLossSpec.Martin  bank_euler_MA=10  bank_heat_coeff_spec_MA=fluids.interfaces.heat_exchangers.enum.BankHeatCoeffSpec.Martin  bank_colburn_coeff_MA=[.27, .63, .36]  generic_flow_area_MA=evaporator_air_min_flow_area m^2  generic_heat_area_MA=evaporator_ht_surf_area_without_fins m^2  generic_volume_MA=evaporator_air_min_flow_area*radiator_tube_width m^3  generic_loss_coeff_MA=evaporator_air_pressure_loss_coef  generic_colburn_coeff_MA=evap_air_side_coef  fouling_factor_MA=0 K*m^2/kW  fin_area_MA=evaporator_fin_surf_area m^2  fin_efficiency_MA=evaporator_air_fin_eff  p_init_MA=ambient_pressure MPa  T_init_MA=ambient_temp K  moisture_spec_MA=foundation.enum.moisture_spec.relative_humidity  RH_init_MA=ambient_rh  x_w_init_MA=0.01  y_w_init_MA=0.01  HR_init_MA=0.01  trace_gas_spec_MA=foundation.enum.trace_gas_spec.mole_fraction  x_g_init_MA=ambient_co2  y_g_init_MA=ambient_co2  RH_ws_MA=1
      settings: SourceProductBaseCode=SH  InternalSimscapePortConfiguration="{\"Bottom\":[],\"Left\":[{\"id\":\"A1\",\"label\":\"A1\",\"type\":\"foundation.thermal_liquid.thermal_liquid\"},{\"id\":\"B1\",\"label\":\"B1\",\"type\":\"foundation.thermal_liquid.thermal_liquid\"}],\"Right\":[{\"id\":\"A2\",\"label\":\"A2\",\"type\":\"foundation.moist_air.moist_air\"},{\"id\":\"B2\",\"label\":\"B2\",\"type\":\"foundation.moist_air.moist_air\"}],\"Top\":[{\"id\":\"W\",\"label\":\"W\",\"type\":\"output\"}]}"
  MA In : PMIOPort  Side=Left
  MA Out : PMIOPort  Port=2  Side=Left
  Coolant out : PMIOPort  Port=3  Side=Right
  Coolant in : PMIOPort  Port=4  Side=Right
  tag scope: T_air_evap_out=global
  wires:
  Sign/1 -> Product/2
  Transfer Fcn/1 -> Max Flow [m^3/s]/1
  Sum1/1 -> Sign/1
  PID Controller/1 -> Transfer Fcn/1
  Product/1 -> PID Controller/1
  [T_cabin] -> Sum/2
  Constant/1 -> Sum1/1, Sum/1
  Sum/1 -> Product/1
  Constant1/1 -> Sum1/2
  Max Flow [m^3/s]/1 -> Scope/1
  PS-Simulink Converter4/1 -> [T_air_evap_out]
  Air Flow Rate1/1 -> Simulink-PS Converter9/1
  connections:
  MA In/RConn1 -- Controlled Volumetric Flow Rate Source (MA)/LConn1
  cabin_hx/RConn2 -- Pressure & Temperature Sensor (MA)1/LConn1 -- MA Out/RConn1
  cabin_hx/LConn1 -- Coolant in/RConn1
  Simulink-PS Converter9/RConn1 -- Controlled Volumetric Flow Rate Source (MA)/LConn2
  cabin_hx/RConn1 -- Controlled Volumetric Flow Rate Source (MA)/RConn1
  cabin_hx/LConn2 -- Coolant out/RConn1
  PS-Simulink Converter4/LConn1 -- Pressure & Temperature Sensor (MA)1/RConn3
  Absolute Reference (MA)1/LConn1 -- Pressure & Temperature Sensor (MA)1/RConn1
